simulink model "ALL_JP360_DBW_V6_5_1103"  (R2022a)
settings: Solver=FixedStepAuto  StartTime=0.0  StopTime=inf  FixedStep=0.01  RelTol=1e-3  EnableMultiTasking=on
model workspace (MAT data in the model file):
  g = 9.8
undefined symbols (not defined in the file or in its folder): canChannel, delta_v_p, IPM_Line_C0, IPM_Line_C1, IPM_Line_C2, IPM_Line_C3, M, M_p, MRR_ObjDistX, MRR_ObjDistY, MRR_ObjFusionCamID, MRR_ObjFusionSig, MRR_ObjID, MRR_ObjRelVelX, MRR_ObjRelVelY, MRR_ObjType, MRR_ObjUpdFlg, none, obj_vaild, untracktime, V, videoinput
libraries: canfdmsglib x230, canfdlib x76, slpidlib x24, simulink x18, dspstat3 x14, ctrlSharedLib x1, simulink_extras x1, imaqlib x1, realtime_pacer_lib x1, dspvision x1, visionsinks x1
(part 2 of 55)

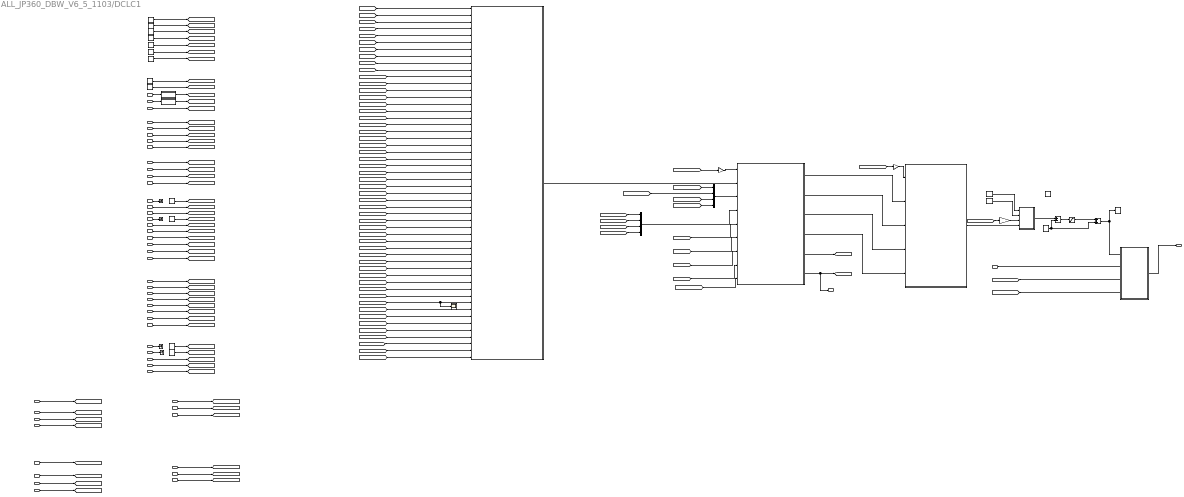
== system ALL_JP360_DBW_V6_5_1103/DCLC1 ==
  note: 0x0: Undecided 0x1: Solid实线 0x2: Road Edge道路边缘 0x3: Dashed虚线 0x4: Double 双线 0x5: Bott's Dots美国特有的凸点标线
  note: 0: OFF 1: PASSIVE/STANDBY 4: ACTIVE 5: ERROR
  note: 0: OFF 1: Passive 2: Stand-By 3: Active-Control 5: Override 6:Standstill 7:Failure
  note: 参数权重
  note: DCLC
      | 使能信号
  note: 刹车油门
      | 转向灯方向盘
  note: 自车速度、加速度
  note: 车道线
  note: 车道线系数
  note: 1V1R
  note: 左前
  note: 右前
  note: 左后
  note: 右后
  ACC_Enable : Inport
  LKA_Enable : Inport  Port=2
  DCLC_Enable : Inport  Port=3  OutDataTypeStr=boolean
  ESP_Algt : Inport  Port=4
  ESP_Alat : Inport  Port=5
  ABS_VehSpdLgt : Inport  Port=6  OutDataTypeStr=single
  ABS_VehSpdLat : Inport  Port=7
  Obj_Speed : Inport  Port=8  OutDataTypeStr=single
  FLR_ObjRelVel : Inport  Port=9
  FLR_OBJ1_Dx : Inport  Port=10
  FLR_OBJ1_Dy : Inport  Port=11
  FRR_ObjRelVel : Inport  Port=12
  FRR_SystemStatus : Inport  Port=13
  FRR_OBJ1_Dx : Inport  Port=14
  FRR_OBJ1_Dy : Inport  Port=15
  RRR_ObjRelVel : Inport  Port=16
  RRR_SystemStatus : Inport  Port=17
  RRR_OBJ1_Dx : Inport  Port=18
  RRR_OBJ1_Dy : Inport  Port=19
  RLR_ObjRelVel : Inport  Port=20
  RLR_OBJ1_Dx : Inport  Port=21
  RLR_OBJ1_Dy : Inport  Port=22
  EMS_BrkPedalStasus : Inport  Port=23
  EMS_AccRAWPedalRatio : Inport  Port=24
  BCM_TurnIndicatorSts : Inport  Port=25
  BCM_TurnIndicatorDig : Inport  Port=26
  EPS_TorsionBarTorque : Inport  Port=27  OutDataTypeStr=single
  IPM_SensorState : Inport  Port=28
  IPM_Line01_ColorClass : Inport  Port=29
  IPM_Line01_Type : Inport  Port=30
  IPM_Line01_C2 : Inport  Port=31  OutDataTypeStr=single
  IPM_Line02_ColorClass : Inport  Port=32
  IPM_Line02_Type : Inport  Port=33
  IPM_Line02_C2 : Inport  Port=34  OutDataTypeStr=single
  IPM_Line01_C0 : Inport  Port=35  OutDataTypeStr=single
  IPM_Line02_C0 : Inport  Port=36  OutDataTypeStr=single
  IPM_Line03_C0 : Inport  Port=37  OutDataTypeStr=single
  IPM_Line04_C0 : Inport  Port=38  OutDataTypeStr=single
  IPM_Line01_C1 : Inport  Port=39  OutDataTypeStr=single
  IPM_Line02_C1 : Inport  Port=40  OutDataTypeStr=single
  IPM_Line03_C1 : Inport  Port=41  OutDataTypeStr=single
  IPM_Line04_C1 : Inport  Port=42  OutDataTypeStr=single
  IPM_Line01_Existence_Probability : Inport  Port=43  OutDataTypeStr=single
  IPM_Line02_Existence_Probability : Inport  Port=44  OutDataTypeStr=single
  MRR_F_Object_dx : Inport  Port=45  OutDataTypeStr=single
  MRR_F_Object_dy : Inport  Port=46  OutDataTypeStr=single
  MRR_HWFail : Inport  Port=47
  IPM_Line03_Existence_Probability : Inport  Port=48  OutDataTypeStr=single
  IPM_Line04_Existence_Probability : Inport  Port=49  OutDataTypeStr=single
  SAS_SteerWheelAngle1 : Inport  Port=50
  Add : Sum  Inputs=+-
  Add1 : Sum
  AngleSaftyLimitedCal : MATLAB Function  TreatAsAtomicUnit=on
  Constant : Constant  Value=0.5  OutDataTypeStr=single
  Constant1 : Constant  Value=2.8  OutDataTypeStr=single
  Constant11 : Constant  Value=1.5  OutDataTypeStr=single
  Constant12 : Constant  Value=200  OutDataTypeStr=int32
  Constant13 : Constant  Value=100  OutDataTypeStr=single
  Constant2 : Constant
  Constant3 : Constant
  Constant{36..37,41,45} (4 alike) : Constant  OutDataTypeStr=single
  Constant4 : Constant  Value=100
  Constant48 : Constant  Value=130  OutDataTypeStr=single
  Constant49 : Constant  Value=20  OutDataTypeStr=single
  Constant5 : Constant  Value=150
  DCLC planner : Subsystem
  DCLC状态机 : Subsystem
  Data Store Memory : DataStoreMemory  DataStoreName=angle  ReadBeforeWriteMsg=warning  WriteAfterWriteMsg=warning  WriteAfterReadMsg=warning  ShowAdditionalParam=off  OutDataTypeStr=single
  Data Store Read : DataStoreRead  DataStoreName=angle  IndexOptions=Index vector (dialog)  Indices=1  OutputSizes=1
  Data Store Write : DataStoreWrite  DataStoreName=angle  IndexOptions=Index vector (dialog)  Indices=1  OutputSizes=1
  Gain1 : Gain  Gain=1/3.6
  Gain2 : Gain  Gain=1/3.6
  Gain3 : Gain  Gain=1/3.6
  LQR : Subsystem
  MATLAB Function : MATLAB Function  TreatAsAtomicUnit=on
  MATLAB Function1 : MATLAB Function  TreatAsAtomicUnit=on
  Mux : Mux
  Mux1 : Mux
  Saturation : Saturate  UpperLimit=0.1  LowerLimit=-0.1
  Scope : Scope
  Terminator{,1..3} (4 alike) : Terminator
  steering_angle_to_torque : Subsystem
  torque : Outport
  DCLC_status : Outport  Port=2
  wires:
  [ESP_Alat] -> DCLC状态机/10(ay)  "自车加速度 ay"
  FLR_OBJ1_Dy/1 -> [FLR_OBJ1_Dy]
  [FRR_ObjRelVel] -> DCLC状态机/6(右前车速度m/s)  "右前车速度m/s"
  [EPS_TorsionBarTorque] -> DCLC状态机/17(方向盘手力矩)  "方向盘手力矩"
  IPM_Line04_C1/1 -> [IPM_Line04_C1]
  Mux/1 -> DCLC planner/3(c0)  "c0"
  [FRR_OBJ1_Dy] -> DCLC状态机/42(与右前车的距离的y)  "与右前车的距离的y"
  [BCM_TurnIndicatorDig] -> DCLC状态机/16(转向灯故障)  "转向灯故障"
  [IPM_Line02_C2] -> DCLC状态机/49(右车道线曲率)  "左车道线的曲率"
  [ACC_Enable] -> DCLC状态机/45(ACC激活信号（暂定为1）)  "ACC激活信号（暂定为1）"
  [ABS_VehSpdLat] -> DCLC状态机/12(vy)  "自车速度 vy 暂定为0"
  [IPM_Line02_C0] -> DCLC状态机/24(后轴中心到右车道线的横向距离)  "后轴中心到右车道线的横向距离"
  DCLC planner/3(theta) -> LQR/4(thetar)  "theta"
  RRR_OBJ1_Dy/1 -> [RRR_OBJ1_Dy]
  EMS_AccRAWPedalRatio/1 -> [EMS_AccRAWPedalRatio]
  [t_lc] -> DCLC状态机/3(t_lc)  "t_lc"
  [IPM_Line04_C0] -> Mux/4
  [DCLC_Enable] -> DCLC状态机/43(DCLC开关)  "DCLC开关"
  RRR_ObjRelVel/1 -> [RRR_ObjRelVel]
  DCLC planner/5(reach_dest) -> [Reach_Destination]
  [DCLC_Speed_Upper] -> DCLC状态机/35(DCLC失效车速上限/km/h)  "DCLC失效车速上限/km/h"
  [ESP_Algt] -> DCLC状态机/9(ax)  "自车加速度 ax"
  [RLR_ObjRelVel] -> DCLC状态机/8(左后车速度m/s)  "左后车速度m/s"
  [IPM_Line03_C0] -> Mux/1
  [t_headway] -> DCLC状态机/1(t_headway)  "t_headway"
  [FRR_SystemStatus] -> DCLC状态机/19(右前雷达状态)  "右前雷达状态"
  IPM_Line02_Type/1 -> [IPM_Line02_Type]
  [IPM_Line01_Type] -> DCLC状态机/21(左车道线类型)  "左车道线类型"
  DCLC planner/2(yrr) -> LQR/3(yrr)  "yrr"
  RRR_SystemStatus/1 -> [RRR_SystemStatus]
  [IPM_Line01_Existence_Probability] -> DCLC状态机/37(左车道清晰状态（信号名暂不确定）)  "左车道清晰状态（信号名暂不确定）"
  [IPM_SensorState] -> DCLC状态机/25(摄像头状态)  "摄像头状态"
  LKA_Enable/1 -> MATLAB Function1/1(LKA_Enable)
  [ABS_VehSpdLgt] -> Gain2/1  "vx"
  [IPM_Line02_ColorClass] -> DCLC状态机/47(右车道线颜色)  "右车道线颜色"
  [Reach_Destination] -> Scope/1, DCLC状态机/44(换道结束标志（DCLC算法给出）)  "换道结束标志（DCLC算法给出）"
  [MRR_HWFail] -> DCLC状态机/28(1V1R雷达故障)  "1V1R雷达故障"
  [IPM_Line02_C1] -> Mux1/3
  DCLC planner/4(kr) -> LQR/5(kappar)  "kr"
  [FRR_OBJ1_Dx] -> DCLC状态机/41(与右前车的距离的x)  "与右前车的距离的x"
  DCLC状态机/1(dclc_sts) -> DCLC planner/2(dclc_sts)  "dclc_sts"
  [t_del] -> DCLC状态机/2(t_del)  "t_del"
  [BCM_TurnIndicatorSts] -> DCLC状态机/15(转向灯请求)  "转向灯请求"
  [lat_weight] -> DCLC planner/7(lat_weight)
  [IPM_Line01_ColorClass] -> DCLC状态机/20(左车道线颜色)  "左车道线颜色"
  [MRR_F_Object_dy] -> DCLC状态机/27(与前车的距离的y)  "与前车的距离的y"
  [EMS_AccRAWPedalRatio] -> DCLC状态机/14(油门信号有效性)  "油门信号有效性"
  [Obj_Speed] -> DCLC状态机/4(前车速度m/s)  "前车速度m/s"
  [IPM_Line01_C0] -> DCLC状态机/22(后轴中心到左车道线的横向距离)  "后轴中心到左车道线的横向距离"
  [RLR_OBJ1_Dx] -> DCLC状态机/29(与左后车的距离的x)  "与左后车的距离的x"
  [FLR_OBJ1_Dx] -> DCLC状态机/39(与左前车的距离的x)  "与左前车的距离的x"
  [RRR_OBJ1_Dx] -> DCLC状态机/32(与右后车的距离的x)  "与右后车的距离的x"
  BCM_TurnIndicatorSts/1 -> [BCM_TurnIndicatorSts]
  [ABS_VehSpdLgt] -> DCLC状态机/11(vx)  "自车速度 vx"
  [FRR_SystemStatus] -> DCLC状态机/18(左前雷达故障（用右前代替）)  "左前雷达故障（用右前代替）"
  [EMS_BrkPedalStasus] -> DCLC状态机/13(刹车信号有效性)  "刹车信号有效性"
  DCLC planner/1(xrr) -> LQR/2(xrr)  "xrr"
  [IPM_Line01_C0] -> Mux/2
  [MRR_F_Object_dx] -> DCLC状态机/26(与前车的距离的x)  "与前车的距离的x"
  [FLR_OBJ1_Dy] -> DCLC状态机/40(与左前车的距离的y)  "与左前车的距离的y"
  [pre_positio] -> DCLC planner/5(start_position)
  MRR_F_Object_dy/1 -> [MRR_F_Object_dy]
  [IPM_Line02_Existence_Probability] -> DCLC状态机/38(右车道清晰状态（信号名暂不确定）)  "右车道清晰状态（信号名暂不确定）"
  [LKA_Enable] -> DCLC状态机/46(LKA激活信号（暂定为1）)  "LKA激活信号（暂定为1）"
  [RLR_OBJ1_Dy] -> DCLC状态机/30(与左后车的距离的y)  "与左后车的距离的y"
  [DCLC_Speed_Lower] -> DCLC状态机/36(DCLC失效车速下限/km/h)  "DCLC失效车速下限/km/h"
  [RRR_SystemStatus] -> DCLC状态机/34(右后雷达状态)  "右后雷达状态"
  [RRR_ObjRelVel] -> DCLC状态机/7(右后车速度m/s)  "右后车速度m/s"
  [IPM_Line01_C2] -> DCLC状态机/23(左车道线的曲率)  "左车道线的曲率"
  [IPM_Line02_C0] -> Mux/3
  [RRR_SystemStatus] -> DCLC状态机/31(左后雷达失效（用右后雷达代替）)  "左后雷达失效（用右后雷达代替）"
  [IPM_Line03_C1] -> Mux1/1
  [IPM_Line01_C1] -> Mux1/2
  [IPM_Line04_C1] -> Mux1/4
  IPM_Line04_C0/1 -> [IPM_Line04_C0]
  [FLR_ObjRelVel] -> DCLC状态机/5(左前车速度m/s)  "左前车速度m/s"
  IPM_Line02_Existence_Probability/1 -> [IPM_Line02_Existence_Probability]
  Mux1/1 -> DCLC planner/4(C1)  "c1"
  [lon_weight] -> DCLC planner/6(lon_weight)
  [IPM_Line02_Type] -> DCLC状态机/48(右车道线类型)  "右车道线类型"
  [RRR_OBJ1_Dy] -> DCLC状态机/33(与右后车的距离的y)  "与右后车的距离的y"
  [change_time_weight] -> DCLC planner/8(change_time_weight)
  FRR_OBJ1_Dx/1 -> [FRR_OBJ1_Dx]
  FRR_ObjRelVel/1 -> [FRR_ObjRelVel]
  MRR_HWFail/1 -> [MRR_HWFail]
  FLR_ObjRelVel/1 -> [FLR_ObjRelVel]
  ABS_VehSpdLat/1 -> [ABS_VehSpdLat]
  IPM_Line01_C1/1 -> [IPM_Line01_C1]
  RLR_OBJ1_Dx/1 -> [RLR_OBJ1_Dx]
  FLR_OBJ1_Dx/1 -> [FLR_OBJ1_Dx]
  ACC_Enable/1 -> MATLAB Function/1(ACC_Enable)
  RLR_ObjRelVel/1 -> [RLR_ObjRelVel]
  FRR_OBJ1_Dy/1 -> [FRR_OBJ1_Dy]
  RRR_OBJ1_Dx/1 -> [RRR_OBJ1_Dx]
  RLR_OBJ1_Dy/1 -> [RLR_OBJ1_Dy]
  FRR_SystemStatus/1 -> [FRR_SystemStatus]
  IPM_Line01_Type/1 -> [IPM_Line01_Type]
  IPM_Line01_Existence_Probability/1 -> [IPM_Line01_Existence_Probability]
  IPM_Line01_C2/1 -> [IPM_Line01_C2]
  IPM_SensorState/1 -> [IPM_SensorState]
  ESP_Algt/1 -> [ESP_Algt]
  EPS_TorsionBarTorque/1 -> [EPS_TorsionBarTorque]
  IPM_Line02_C1/1 -> [IPM_Line02_C1]
  IPM_Line03_C1/1 -> [IPM_Line03_C1]
  ESP_Alat/1 -> [ESP_Alat]
  EMS_BrkPedalStasus/1 -> [EMS_BrkPedalStasus]
  IPM_Line02_C2/1 -> [IPM_Line02_C2]
  IPM_Line03_C0/1 -> [IPM_Line03_C0]
  IPM_Line01_C0/1 -> [IPM_Line01_C0]
  DCLC_Enable/1 -> [DCLC_Enable]
  IPM_Line02_C0/1 -> [IPM_Line02_C0]
  BCM_TurnIndicatorDig/1 -> [BCM_TurnIndicatorDig]
  LQR/1(steering_angle) -> AngleSaftyLimitedCal/4(angle)  "steering_angle"
  Constant/1 -> AngleSaftyLimitedCal/1(a)
  Constant1/1 -> AngleSaftyLimitedCal/2(L)
  [ABS_VehSpdLgt] -> Gain3/1  "vx"
  [ABS_VehSpdLgt] -> Gain1/1
  Gain3/1 -> AngleSaftyLimitedCal/3(V)
  Data Store Read/1 -> Add/2, Add1/2
  Add/1 -> Saturation/1
  Add1/1 -> Data Store Write/1, steering_angle_to_torque/1(desire_steering_angle)
  DCLC planner/6(status) -> DCLC_status/1, [Pass_Midline]
  [Pass_Midline] -> DCLC状态机/50(变道越过车道线标志)  "变道越过车道线标志（1表示未越过车道线，2表示越过车道线）"
  ABS_VehSpdLgt/1 -> [ABS_VehSpdLgt]
  Gain2/1 -> DCLC planner/1(vx)
  Gain1/1 -> LQR/1(vx)
  Constant41/1 -> [t_del]
  Constant12/1 -> [pre_positio]
  Constant36/1 -> [lon_weight]
  Constant13/1 -> [lat_weight]
  Constant37/1 -> [change_time_weight]
  Constant45/1 -> [t_lc]
  Constant11/1 -> [t_headway]
  Constant49/1 -> [DCLC_Speed_Lower]
  Constant48/1 -> [DCLC_Speed_Upper]
  IPM_Line01_ColorClass/1 -> Terminator/1
  Constant2/1 -> [IPM_Line01_ColorClass]
  IPM_Line02_ColorClass/1 -> Terminator1/1
  Constant3/1 -> [IPM_Line02_ColorClass]
  Obj_Speed/1 -> Terminator2/1
  Constant4/1 -> [Obj_Speed]
  MATLAB Function/1(u) -> [ACC_Enable]
  MATLAB Function1/1(u) -> [LKA_Enable]
  IPM_Line03_Existence_Probability/1 -> [IPM_Line03_Existence_Probability]
  IPM_Line04_Existence_Probability/1 -> [IPM_Line04_Existence_Probability]
  [IPM_Line03_Existence_Probability] -> DCLC状态机/51(leftleft_line_pro)  "左左车道线清晰状态"
  [IPM_Line04_Existence_Probability] -> DCLC状态机/52(rightright_line_pro)  "右右车道线清晰状态"
  MRR_F_Object_dx/1 -> Terminator3/1
  Constant5/1 -> [MRR_F_Object_dx]
  AngleSaftyLimitedCal/1(angle_limited) -> Add/1
  Saturation/1 -> Add1/1
  [ABS_VehSpdLgt] -> steering_angle_to_torque/3(vx km/h)
  SAS_SteerWheelAngle1/1 -> steering_angle_to_torque/2(acture_steering_angle)
  [ABS_VehSpdLat] -> steering_angle_to_torque/4(vy km/h)
  steering_angle_to_torque/1(torque) -> torque/1
  [BCM_TurnIndicatorSts] -> DCLC planner/9(turn_request)  "转向灯请求"

== system ALL_JP360_DBW_V6_5_1103/Error ==

== system ALL_JP360_DBW_V6_5_1103/LKA_Control ==
  note: 0: OFF
      | 1: Passive
      | 2: Stand-By
      | 3: Active-Control
      | 5: Override
      | 6: Standstill
      | 7: Failure
  note: Lane_status:
      | 0：无车道线
      | 1：单车道线
      | 2：双车道线
      | 3：骑线
  SWM : Inport
  SWM_TurnIndicatorAct : Inport  Port=2
  ESP_YawRateStatus : Inport  Port=3
  ABS_VehSpdLgtStatus : Inport  Port=4
  ESP_Master_Cylinder_Pressure : Inport  Port=5
  SRS_SBR_Driver : Inport  Port=6
  MRR_HWFail : Inport  Port=7
  IPM_SensorState : Inport  Port=8
  TCU_GearSelectorReq : Inport  Port=9
  SAS_SteerWheelRotSpd : Inport  Port=10
  EPS_TorsionBarTorque : Inport  Port=11
  ESP_EspCtrlActv : Inport  Port=12
  EMS_IndicatedEngError : Inport  Port=13
  BCM_DoorStsFrntLe : Inport  Port=14
  BCM_DoorStsRearRi : Inport  Port=15
  BCM_DoorStsFrntRi : Inport  Port=16
  BCM_DoorStsRearLe : Inport  Port=17
  BCM_EnginehoodSts : Inport  Port=18
  ESP_YawRate : Inport  Port=19
  ABS_VehSpdLgt : Inport  Port=20
  ABS_AbsCtrlActv : Inport  Port=21
  SAS_SteerWheelAngle : Inport  Port=22
  SAS_SteerWheelRotSpdStatus : Inport  Port=23
  EPS_LKAControlStatus : Inport  Port=24
  EPS_LKAResponseTorque : Inport  Port=25
  EPS_EPSPAMSts : Inport  Port=26
  ESP_EspEnableSts : Inport  Port=27
  ESP_Master_Cylinder_Pressure_Status : Inport  Port=28
  IPM_Line01_C0 : Inport  Port=29
  IPM_Line01_C1 : Inport  Port=30
  IPM_Line01_C2 : Inport  Port=31
  IPM_Line01_C3 : Inport  Port=32
  IPM_Line02_C0 : Inport  Port=33
  IPM_Line02_C1 : Inport  Port=34
  IPM_Line02_C2 : Inport  Port=35
  IPM_Line02_C3 : Inport  Port=36
  IPM_Line01_Existence_Probability : Inport  Port=37
  IPM_Line02_Existence_Probability : Inport  Port=38
  acc_sta : Inport  Port=39
  DCLC_Status : Inport  Port=40
  Chart : Stateflow chart  TreatAsAtomicUnit=on
  Constant : Constant  Value=0  OutDataTypeStr=int8
  Constant1 : Constant  Value=3  OutDataTypeStr=single
  Constant3 : Constant  Value=0  OutDataTypeStr=int8
  Constant5 : Constant  OutDataTypeStr=int8
  Data Type Conversion : DataTypeConversion  OutDataTypeStr=single  SaturateOnIntegerOverflow=off  RndMeth=Floor
  Data Type Conversion3 : DataTypeConversion  OutDataTypeStr=int8  SaturateOnIntegerOverflow=off  RndMeth=Floor
  Display{,1..4} (5 alike) : Display
  LKA_Cal : Subsystem
  Lane_Status : Subsystem
  Mux1 : Mux  Inputs=8
  Scope : Scope  NumInputPorts=2
  To Workspace : ToWorkspace  VariableName=L_status  SaveFormat=Timeseries  SampleTime=-1
  To Workspace1 : ToWorkspace  VariableName=LKA_status  SaveFormat=Structure With Time  SampleTime=-1
  To Workspace2 : ToWorkspace  VariableName=TorsionBar_tor  SaveFormat=Structure With Time  SampleTime=-1
  To Workspace3 : ToWorkspace  VariableName=C  SaveFormat=Structure With Time  SampleTime=-1
  To Workspace4 : ToWorkspace  VariableName=L1_pro  SaveFormat=Structure With Time  SampleTime=-1
  To Workspace5 : ToWorkspace  VariableName=L2_pro  SaveFormat=Structure With Time  SampleTime=-1
  LKAReq_angle : Outport
  IPM_LineAssit_Status : Outport  Port=2
  err_now : Outport  Port=3
  wires:
  ESP_Master_Cylinder_Pressure_Status/1 -> Chart/33(ESP_Master_Cylinder_Pressure_Status)
  BCM_DoorStsRearLe/1 -> Chart/20(BCM_DoorStsRearLe)
  ESP_EspCtrlActv/1 -> Chart/26(ESP_EspCtrlActv)
  EPS_EPSPAMSts/1 -> Chart/29(EPS_EPSPAMSts)
  [ABS_VehSpdLgt] -> LKA_Cal/4(ABS_Vhlspd)
  SRS_SBR_Driver/1 -> Chart/21(SRS_SBR_Driver)
  BCM_DoorStsFrntRi/1 -> Chart/19(BCM_DoorStsFrntRi)
  [C2] -> Chart/9(LaneCurvature)
  BCM_DoorStsFrntLe/1 -> Chart/17(BCM_DoorStsFrntLe)
  EPS_TorsionBarTorque/1 -> To Workspace2/1, Chart/24(EPS_TorsionBarTorque), Display/1
  EPS_LKAResponseTorque/1 -> Chart/28(EPS_LKAResponseTorque)
  EPS_LKAControlStatus/1 -> Chart/25(EPS_LKAControlStatus)
  EMS_IndicatedEngError/1 -> Chart/30(EMS_IndicatedEngError)
  Data Type Conversion3/1 -> Chart/5(ESP_YawRateStatus)
  Constant5/1 -> Chart/2(IPM_LineAssit_LeftVisualization), Chart/3(IPM_LineAssit_RightVisualization)
  TCU_GearSelectorReq/1 -> Chart/23(TCU_GearSelectorReq)
  SAS_SteerWheelRotSpd/1 -> Chart/27(SAS_SteerWheelRotSpd)
  ESP_YawRateStatus/1 -> Data Type Conversion3/1
  ESP_YawRate/1 -> Chart/6(ESP_YawRate)
  BCM_DoorStsRearRi/1 -> Chart/18(BCM_DoorStsRearRi)
  BCM_EnginehoodSts/1 -> Chart/22(BCM_EnginehoodSts)
  SAS_SteerWheelRotSpdStatus/1 -> Chart/32(SAS_SteerWheelRotSpdStatus)
  Constant3/1 -> Chart/11(LaneChange)
  IPM_SensorState/1 -> Chart/14(IPM_SensorState)
  Chart/1(IPM_LineAssit_Status) -> Display3/1, To Workspace1/1, Scope/2, [LKA_status], IPM_LineAssit_Status/1  "LKA"
  ABS_AbsCtrlActv/1 -> Chart/12(ABS_AbsCtrlActv)
  SAS_SteerWheelAngle/1 -> LKA_Cal/3(SAS_SteerWheelAngle), Display2/1
  ESP_EspEnableSts/1 -> Chart/31(ESP_EspEnableSts)
  MRR_HWFail/1 -> Chart/13(MRR_HWFail)
  ABS_VehSpdLgt/1 -> Data Type Conversion/1, [ABS_VehSpdLgt]
  ABS_VehSpdLgtStatus/1 -> Chart/7(ABS_VehSpdLgtStatus)
  Constant/1 -> Chart/15(lka_state_sw)
  Data Type Conversion/1 -> Chart/8(ABS_VehSpdLgt)
  [Ct] -> LKA_Cal/1(Ct)
  Constant1/1 -> Chart/10(LaneWidth)
  ESP_Master_Cylinder_Pressure/1 -> Chart/16(ESP_Master_Cylinder_Pressure)
  SWM/1 -> Chart/1(LKASwitch)
  IPM_Line01_Existence_Probability/1 -> Lane_Status/2(IPM_Line01_Existence_Probability), To Workspace4/1
  IPM_Line02_Existence_Probability/1 -> Lane_Status/3(IPM_Line02_Existence_Probability), To Workspace5/1
  Lane_Status/1(Ct) -> [Ct]
  Lane_Status/2(lane_status) -> Scope/1, [Lane_status], Display1/1, To Workspace/1  "lane"
  [Lane_status] -> Chart/34(Lane_status)
  SWM_TurnIndicatorAct/1 -> Chart/4(SWM_TurnIndicationAct)
  LKA_Cal/1(LKAReq_angle) -> LKAReq_angle/1, Display4/1
  DCLC_Status/1 -> Chart/35(DCLC_Status)
  acc_sta/1 -> Chart/36(acc_sta)
  Lane_Status/3(ang) -> [ang]
  [ang] -> Chart/37(degre)
  LKA_Cal/2(err_now) -> err_now/1
  [LKA_status] -> LKA_Cal/2(LKA_status)
  Lane_Status/4(C2) -> [C2]
  Mux1/1 -> Lane_Status/1(LRC), To Workspace3/1
  IPM_Line01_C0/1 -> Mux1/1
  IPM_Line01_C1/1 -> Mux1/2
  IPM_Line01_C2/1 -> Mux1/3
  IPM_Line02_C0/1 -> Mux1/5
  IPM_Line02_C1/1 -> Mux1/6
  IPM_Line01_C3/1 -> Mux1/4
  IPM_Line02_C2/1 -> Mux1/7
  IPM_Line02_C3/1 -> Mux1/8

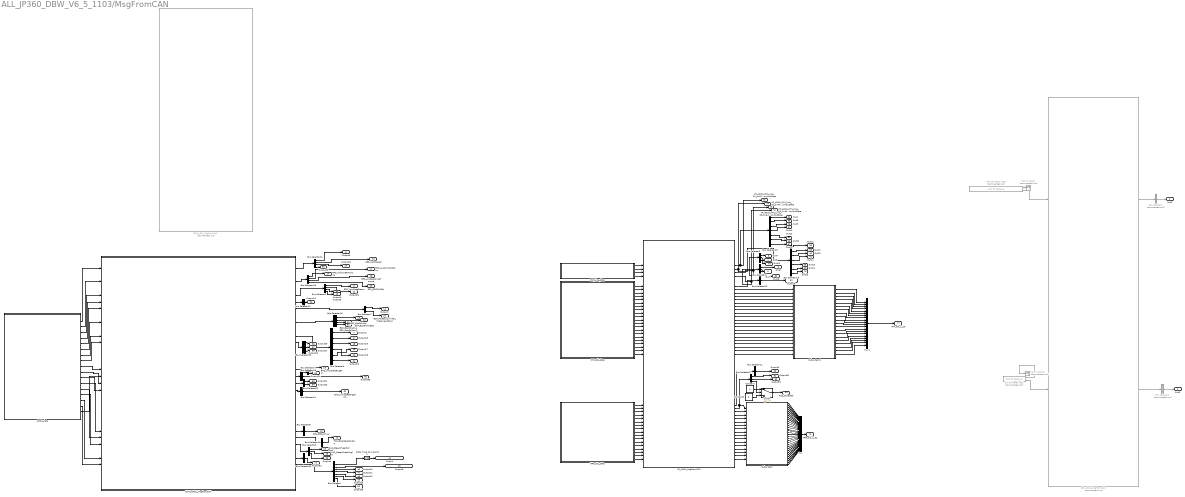
== system ALL_JP360_DBW_V6_5_1103/MsgFromCAN ==
  ADCU_data : Subsystem
  Bus Selector : BusSelector  OutputSignals=SWM_LaneAssistSwitch,SWM_ACCResume,SWM_ACCSet,SWM_ACCSwitch,SWM_ACCvSetPlus,SWM_ACCvSetMinus,SWM_ACCtauGapSetMinus
  Bus Selector1 : BusSelector  Commented=on  OutputSignals=FRR_SystemStatus
  Bus Selector10 : BusSelector  OutputSignals=IPM_SensorState
  Bus Selector11 : BusSelector  OutputSignals=MRR_HWFail
  Bus Selector12 : BusSelector  OutputSignals=ABS_VehSpdLgtStatus,ABS_VehSpdLgt,ABS_AbsCtrlActv,ABS_VehSpdDirection
  Bus Selector13 : BusSelector  OutputSignals=IPM_Line01_C0,IPM_Line01_C1,IPM_Line01_C2,IPM_Line01_C3,IPM_Line01_Type,IPM_Line01_ColorClass,IPM_Line01_Existence_Probability
  Bus Selector14 : BusSelector  OutputSignals=TCU_GearSelectorReq
  Bus Selector15 : BusSelector  OutputSignals=EPS_TorsionBarTorque,EPS_LKAControlStatus,EPS_LKAResponseTorque,EPS_EPSPAMSts
  Bus Selector16 : BusSelector  OutputSignals=ESP_EspCtrlActv,ESP_EspEnableSts,ESP_EPBStatus,ESP_AvhActive
  Bus Selector17 : BusSelector  OutputSignals=EMS_IndicatedEngError,EMS_IndicatedDriverOverride
  Bus Selector18 : BusSelector  OutputSignals=IPM_Line02_C0,IPM_Line02_C1,IPM_Line02_C2,IPM_Line02_C3,IPM_Line02_Type,IPM_Line02_ColorClass,IPM_Line02_Existence_Probability
  Bus Selector19 : BusSelector  OutputSignals=EMS_IndicatedRealEngTorq
  Bus Selector2 : BusSelector  Commented=on  OutputSignals=RRR_SystemStatus
  Bus Selector21 : BusSelector  OutputSignals=ESP_VehicleStandstill
  Bus Selector22 : BusSelector  OutputSignals=EMS_AccRAWPedalRatio,EMS_BrkPedalStasus
  Bus Selector23 : BusSelector  OutputSignals=BCM_PowerModeInvalid,BCM_PowerMode,BCM_Mechanical_Hand_Brake
  Bus Selector24 : BusSelector  OutputSignals=IC_VehSpd_HMI
  Bus Selector27 : BusSelector  OutputSignals=MRR_ObjDistX_01,MRR_ObjRelVelX_01,MRR_ObjType_01
  Bus Selector28 : BusSelector  OutputSignals=SWM_TurnIndicationAct
  Bus Selector3 : BusSelector  OutputSignals=IPM_Line03_C0,IPM_Line03_C1,IPM_Line03_Existence_Probability
  Bus Selector4 : BusSelector  OutputSignals=IPM_Line04_C0,IPM_Line04_C1,IPM_Line04_Existence_Probability
  Bus Selector5 : BusSelector  OutputSignals=ESP_YawRateStatus,ESP_YawRate,ESP_Alat,ESP_Algt
  Bus Selector6 : BusSelector  OutputSignals=BCM_TurnIndicatorSts,BCM_DoorStsFrntLe,BCM_DoorStsRearRi,BCM_DoorStsRearLe,BCM_DoorStsFrntRi,BCM_EnginehoodSts
  Bus Selector7 : BusSelector  OutputSignals=ESP_Master_Cylinder_Pressure,ESP_Master_Cylinder_Pressure_Status
  Bus Selector8 : BusSelector  OutputSignals=SRS_SBR_Driver
  Bus Selector9 : BusSelector  OutputSignals=SAS_SteerWheelRotSpd,SAS_SteerWheelAngle,SAS_SteerWheelRotSpdStatus
  CAN FD Receive50 : canfdlib/CAN FD Receive  Commented=on  BlockHandle=78400.0006  Device=MathWorks Virtual 1 (Channel 1)  ObjConstructor=canChannel('MathWorks', 'Virtual 1', 1, 'ProtocolMode', 'CAN FD')  EnableStandardIDsFilter=off  StdIDsCombo=Allow only  StandardIDs=114  EnableExtendedIDsFilter=off  ExtIDsCombo=Allow all  ExtendedIDs=0  SampleTime=0.01  MsgsPerTimestep=all  InternalFilterUpdateStatus=on  BusOutput=on
      settings: SourceProductBaseCode=VN
  CAN FD Receive51 : canfdlib/CAN FD Receive  Commented=on  BlockHandle=78403.0004  Device=MathWorks Virtual 1 (Channel 1)  ObjConstructor=canChannel('MathWorks', 'Virtual 1', 1, 'ProtocolMode', 'CAN FD')  EnableStandardIDsFilter=off  StdIDsCombo=Allow only  StandardIDs=115  EnableExtendedIDsFilter=off  ExtIDsCombo=Allow all  ExtendedIDs=0  SampleTime=0.01  MsgsPerTimestep=all  InternalFilterUpdateStatus=on  BusOutput=on
      settings: SourceProductBaseCode=VN
  CCAN_ADCU_MsgFromCAN : Subsystem
  CCAN_GW_MsgFromCAN : Subsystem  Commented=on
  Constant : Constant  OutDataTypeStr=boolean
  Constant1 : Constant  Value=0  OutDataTypeStr=boolean
  Data Type Conversion1 : DataTypeConversion  OutDataTypeStr=int8  SaturateOnIntegerOverflow=off  RndMeth=Floor
  IPM_Line_data : Subsystem
  IPM_Obj_data : Subsystem
  MRR_Obj_data : Subsystem
  Mux : Mux  Inputs=32
  Mux1 : Mux  Inputs=20
  SRR_ADCU_MsgFromCAN : Subsystem  Commented=on
  Subsystem : Subsystem
  Subsystem1 : Subsystem
  Switch : Switch  Criteria=u2 > Threshold  SaturateOnIntegerOverflow=off  InputSameDT=off
  Terminator22 : Terminator  Commented=on
  Terminator23 : Terminator  Commented=on
  VR_ADCU_MsgFromCAN : Subsystem
  Out2 : Outport
  Out3 : Outport  Port=2
  Out4 : Outport  Port=3
  Out5 : Outport  Port=4
  Out6 : Outport  Port=5
  Out7 : Outport  Port=6
  Output1 : Outport  Port=7
  ESP_YawRateStatus : Outport  Port=8
  Output3 : Outport  Port=9
  SRS_SBR_Driver : Outport  Port=10
  Output7 : Outport  Port=11
  TCU_GearSelectorReq : Outport  Port=12
  SAS_SteerWheelRotSpd : Outport  Port=13
  EPS_TorsionBarTorque : Outport  Port=14
  ESP_EspCtrlActv : Outport  Port=15
  EMS_IndicatedEngError : Outport  Port=16
  Output15 : Outport  Port=17
  Output16 : Outport  Port=18
  Output17 : Outport  Port=19
  Output18 : Outport  Port=20
  Output19 : Outport  Port=21
  Output20 : Outport  Port=22
  ABS_VehSpdLgt : Outport  Port=23
  Output22 : Outport  Port=24
  SAS_SteerWheelAngle : Outport  Port=25
  Output4 : Outport  Port=26
  EPS_LKAControlStatus : Outport  Port=27
  EPS_LKAResponseTorque : Outport  Port=28
  EPS_EPSPAMSts : Outport  Port=29
  ESP_EspEnableSts : Outport  Port=30
  ESP_Master_Cylinder_Pressure_Status : Outport  Port=31
  Output6 : Outport  Port=32
  Output5 : Outport  Port=33
  Out1 : Outport  Port=34
  Out8 : Outport  Port=35
  Out9 : Outport  Port=36
  Out10 : Outport  Port=37
  Out11 : Outport  Port=38
  Out12 : Outport  Port=39
  Out13 : Outport  Port=40
  Out14 : Outport  Port=41
  Output2 : Outport  Port=42
  Output8 : Outport  Port=43
  Output : Outport  Port=44
  Output9 : Outport  Port=45
  Output10 : Outport  Port=46
  Output11 : Outport  Port=47
  Output12 : Outport  Port=48
  Output13 : Outport  Port=49
  Output14 : Outport  Port=50
  ESP_EspCtrlActv1 : Outport  Port=51
  ESP_EspCtrlActv2 : Outport  Port=52
  Output21 : Outport  Port=53
  Output23 : Outport  Port=54
  Output24 : Outport  Port=55
  Output25 : Outport  Port=56
  Output26 : Outport  Port=57
  Output27 : Outport  Port=58
  Output28 : Outport  Port=59
  Output29 : Outport  Port=60
  EMS_IndicatedEngError1 : Outport  Port=61
  Output30 : Outport  Port=62
  Output31 : Outport  Port=63
  ACC_Objected : Outport  Port=64
  Out20 : Outport  Port=65
  Out21 : Outport  Port=66
  Out22 : Outport  Port=67
  Out23 : Outport  Port=68
  Out24 : Outport  Port=69
  Out25 : Outport  Port=70
  Output32 : Outport  Port=71
  MRR_obj_1_32 : Outport  Port=72
  VR_ADCU_IPM_Line_01_0x640FromOutData : Outport  Port=73
  VR_ADCU_IPM_Line_02_0x641FromOutData : Outport  Port=74
  VR_ADCU_IPM_Line_03_0x642FromOutData : Outport  Port=75
  VR_ADCU_IPM_Line_04_0x643FromOutData : Outport  Port=76
  IPM_obj_1_20 : Outport  Port=77
  Output33 : Outport  Port=78
  Out15 : Outport  Port=79
  Out16 : Outport  Port=80
  wires:
  SRR_ADCU_MsgFromCAN/22(SRR_ADCU_FRR_AssistSysSt_0x72FromOutData) -> Bus Selector1/1  "SRR_ADCU_FRR_AssistSysSt_0x72FromOutData"
  Bus Selector1/1 -> Out2/1  "<FRR_SystemStatus>"
  Bus Selector2/1 -> Out3/1  "<RRR_SystemStatus>"
  SRR_ADCU_MsgFromCAN/64(SRR_ADCU_RRR_AssistSysSt_0x73FromOutData) -> Bus Selector2/1  "SRR_ADCU_FRR_AssistSysSt_0x72FromOutData"
  VR_ADCU_MsgFromCAN/8(VR_ADCU_IPM_Line_03_0x642FromOutData) -> VR_ADCU_IPM_Line_03_0x642FromOutData/1, Bus Selector3/1  "VR_ADCU_IPM_Line_03_0x642FromOutData"
  VR_ADCU_MsgFromCAN/9(VR_ADCU_IPM_Line_04_0x643FromOutData) -> Bus Selector4/1, VR_ADCU_IPM_Line_04_0x643FromOutData/1  "VR_ADCU_IPM_Line_04_0x643FromOutData"
  Bus Selector4/1 -> Out6/1  "<IPM_Line04_C0>"
  Bus Selector4/2 -> Out7/1  "<IPM_Line04_C1>"
  Bus Selector3/1 -> Out4/1  "<IPM_Line03_C0>"
  Bus Selector3/2 -> Out5/1  "<IPM_Line03_C1>"
  Bus Selector7/1 -> Output7/1  "<ESP_Master_Cylinder_Pressure>"
  Bus Selector5/2 -> Output20/1  "<ESP_YawRate>"
  Bus Selector7/2 -> ESP_Master_Cylinder_Pressure_Status/1  "<ESP_Master_Cylinder_Pressure_Status>"
  Bus Selector17/1 -> EMS_IndicatedEngError/1  "<EMS_IndicatedEngError>"
  Bus Selector16/2 -> ESP_EspEnableSts/1  "<ESP_EspEnableSts>"
  Bus Selector8/1 -> SRS_SBR_Driver/1  "<SRS_SBR_Driver>"
  Bus Selector12/1 -> Output3/1  "<ABS_VehSpdLgtStatus>"
  Bus Selector15/4 -> EPS_EPSPAMSts/1  "<EPS_EPSPAMSts>"
  CCAN_ADCU_MsgFromCAN/1(CCAN_ADCU_ABS_Sts_0x221FromOutData) -> Bus Selector12/1  "CCAN_ADCU_ABS_Sts_0x221FromOutData"
  Bus Selector9/2 -> SAS_SteerWheelAngle/1  "<SAS_SteerWheelAngle>"
  Bus Selector12/3 -> Output22/1  "<ABS_AbsCtrlActv>"
  CCAN_ADCU_MsgFromCAN/9(CCAN_ADCU_ESP_Status_0x243FromOutData) -> Bus Selector16/1  "CCAN_ADCU_ESP_Status_0x243FromOutData"
  CCAN_ADCU_MsgFromCAN/27(CCAN_ADCU_SAS_Sensor_0x175FromOutData) -> Bus Selector9/1  "CCAN_ADCU_SAS_Sensor_0x175FromOutData"
  Bus Selector6/4 -> Output18/1  "<BCM_DoorStsRearLe>"
  CCAN_ADCU_MsgFromCAN/7(CCAN_ADCU_ESP_Pressure_0x241FromOutData) -> Bus Selector7/1  "CCAN_ADCU_ESP_Pressure_0x241FromOutData"
  CCAN_ADCU_MsgFromCAN/25(CCAN_ADCU_GW_SRS_0x350FromOutData) -> Bus Selector8/1  "CCAN_ADCU_GW_SRS_0x350FromOutData"
  Bus Selector15/3 -> EPS_LKAResponseTorque/1  "<EPS_LKAResponseTorque>"
  Bus Selector6/2 -> Output15/1  "<BCM_DoorStsFrntLe>"
  Bus Selector6/1 -> Output1/1  "<BCM_TurnIndicatorSts>"
  Bus Selector6/6 -> Output19/1  "<BCM_EnginehoodSts>"
  Bus Selector/1 -> Data Type Conversion1/1  "<SWM_LaneAssistSwitch>"
  CCAN_ADCU_MsgFromCAN/26(CCAN_ADCU_GW_TCU_GearInfo_0x123FromOutData) -> Bus Selector14/1  "CCAN_ADCU_GW_TCU_GearInfo_0x123FromOutData"
  CCAN_ADCU_MsgFromCAN/30(CCAN_ADCU_SWM_MRR_0x31BFromOutData) -> Bus Selector/1  "CCAN_ADCU_SWM_MRR_0x31BFromOutData"
  CCAN_ADCU_MsgFromCAN/16(CCAN_ADCU_GW_EMS_TqWhl_0x111FromOutData) -> Bus Selector17/1  "CCAN_ADCU_GW_EMS_TqWhl_0x111FromOutData"
  Bus Selector15/1 -> EPS_TorsionBarTorque/1  "<EPS_TorsionBarTorque>"
  Bus Selector15/2 -> EPS_LKAControlStatus/1  "<EPS_LKAControlStatus>"
  Bus Selector5/1 -> ESP_YawRateStatus/1  "<ESP_YawRateStatus>"
  Bus Selector9/1 -> SAS_SteerWheelRotSpd/1  "<SAS_SteerWheelRotSpd>"
  CCAN_ADCU_MsgFromCAN/5(CCAN_ADCU_ESP_AxAy_0x242FromOutData) -> Bus Selector5/1  "CCAN_ADCU_ESP_AxAy_0x242FromOutData"
  CCAN_ADCU_MsgFromCAN/11(CCAN_ADCU_GW_BCM_Door_0x310FromOutData) -> Bus Selector6/1  "CCAN_ADCU_GW_BCM_Door_0x310FromOutData"
  Bus Selector6/5 -> Output17/1  "<BCM_DoorStsFrntRi>"
  Bus Selector12/2 -> ABS_VehSpdLgt/1  "<ABS_VehSpdLgt>"
  Bus Selector14/1 -> TCU_GearSelectorReq/1  "<TCU_GearSelectorReq>"
  Bus Selector6/3 -> Output16/1  "<BCM_DoorStsRearRi>"
  Bus Selector16/1 -> ESP_EspCtrlActv/1  "<ESP_EspCtrlActv>"
  CCAN_ADCU_MsgFromCAN/3(CCAN_ADCU_EPS_Advanced_0x176FromOutData) -> Bus Selector15/1  "CCAN_ADCU_EPS_Advanced_0x176FromOutData"
  Bus Selector10/1 -> Output6/1  "<IPM_SensorState>"
  VR_ADCU_MsgFromCAN/12(VR_ADCU_IPM_ObjHeader_0x630FromOutData) -> Bus Selector10/1  "VR_ADCU_IPM_ObjHeader_0x630FromOutData"
  Bus Selector11/1 -> Output5/1  "<MRR_HWFail>"
  VR_ADCU_MsgFromCAN/47(VR_ADCU_MRR_ObjHeader_0x680FromOutData) -> Bus Selector11/1  "VR_ADCU_MRR_ObjHeader_0x680FromOutData"
  VR_ADCU_MsgFromCAN/6(VR_ADCU_IPM_Line_01_0x640FromOutData) -> VR_ADCU_IPM_Line_01_0x640FromOutData/1, Bus Selector13/1  "VR_ADCU_IPM_Line_01_0x640FromOutData"
  VR_ADCU_MsgFromCAN/7(VR_ADCU_IPM_Line_02_0x641FromOutData) -> VR_ADCU_IPM_Line_02_0x641FromOutData/1, Bus Selector18/1  "VR_ADCU_IPM_Line_02_0x641FromOutData"
  Bus Selector13/1 -> Out1/1  "<IPM_Line01_C0>"
  Bus Selector13/2 -> Out8/1  "<IPM_Line01_C1>"
  Bus Selector13/3 -> Out9/1  "<IPM_Line01_C2>"
  Bus Selector13/4 -> Out10/1  "<IPM_Line01_C3>"
  Bus Selector18/1 -> Out11/1  "<IPM_Line02_C0>"
  Bus Selector18/2 -> Out12/1  "<IPM_Line02_C1>"
  Bus Selector18/3 -> Out13/1  "<IPM_Line02_C2>"
  Bus Selector18/4 -> Out14/1  "<IPM_Line02_C3>"
  Bus Selector9/3 -> Output4/1  "<SAS_SteerWheelRotSpdStatus>"
  Bus Selector5/3 -> Output2/1  "<ESP_Alat>"
  Bus Selector5/4 -> Output8/1  "<ESP_Algt>"
  Bus Selector/2 -> Output9/1  "<SWM_ACCResume>"
  Bus Selector/3 -> Output10/1  "<SWM_ACCSet>"
  Bus Selector/4 -> Output11/1  "<SWM_ACCSwitch>"
  Bus Selector/5 -> Output12/1  "<SWM_ACCvSetPlus>"
  Bus Selector/6 -> Output13/1  "<SWM_ACCvSetMinus>"
  CCAN_ADCU_MsgFromCAN/6(CCAN_ADCU_ESP_Direction_0x235FromOutData) -> Bus Selector21/1  "CCAN_ADCU_ESP_Direction_0x235FromOutData"
  Bus Selector21/1 -> Output14/1  "<ESP_VehicleStandstill>"
  Bus Selector16/4 -> ESP_EspCtrlActv2/1  "<ESP_AvhActive>"
  Bus Selector16/3 -> ESP_EspCtrlActv1/1  "<ESP_EPBStatus>"
  CCAN_ADCU_MsgFromCAN/18(CCAN_ADCU_GW_EMS_WhlTq_0x107FromOutData) -> Bus Selector22/1  "CCAN_ADCU_GW_EMS_WhlTq_0x107FromOutData"
  Bus Selector22/1 -> Output21/1  "<EMS_AccRAWPedalRatio>"
  Bus Selector22/2 -> Output23/1  "<EMS_BrkPedalStasus>"
  Bus Selector17/2 -> Output24/1  "<EMS_IndicatedDriverOverride>"
  CCAN_ADCU_MsgFromCAN/12(CCAN_ADCU_GW_Body_0x321FromOutData) -> Bus Selector23/1  "CCAN_ADCU_GW_Body_0x321FromOutData"
  Bus Selector23/1 -> Output25/1  "<BCM_PowerModeInvalid>"
  Bus Selector23/2 -> Output26/1  "<BCM_PowerMode>"
  Bus Selector23/3 -> Output27/1  "<BCM_Mechanical_Hand_Brake>"
  Bus Selector12/4 -> Output28/1  "<ABS_VehSpdDirection>"
  Bus Selector/7 -> Output29/1  "<SWM_ACCtauGapSetMinus>"
  CAN FD Receive50/1 -> Terminator22/1
  CAN FD Receive50/2 -> SRR_ADCU_MsgFromCAN/22(SRR_ADCU_FRR_AssistSysSt_0x72FromInData)
  CAN FD Receive51/2 -> SRR_ADCU_MsgFromCAN/64(SRR_ADCU_RRR_AssistSysSt_0x73FromInData)
  CAN FD Receive51/1 -> Terminator23/1
  CCAN_ADCU_MsgFromCAN/19(CCAN_ADCU_GW_IC_0x510FromOutData) -> Bus Selector24/1  "CCAN_ADCU_GW_IC_0x510FromOutData"
  Bus Selector24/1 -> EMS_IndicatedEngError1/1  "<IC_VehSpd_HMI>"
  VR_ADCU_MsgFromCAN/48(VR_ADCU_MRR_Obj_01_02_0x690FromOutData) -> Subsystem/1(VR_ADCU_MRR_Obj_01_02_0x690FromOutData), Bus Selector27/1  "VR_ADCU_MRR_Obj_01_02_0x690FromOutData"
  Bus Selector27/1 -> Output30/1  "<MRR_ObjDistX_01>"
  Bus Selector27/2 -> Output31/1  "<MRR_ObjRelVelX_01>"
  Bus Selector27/3 -> Switch/2  "<MRR_ObjType_01>"
  Constant/1 -> Switch/1
  Constant1/1 -> Switch/3
  Switch/1 -> ACC_Objected/1
  Bus Selector13/5 -> Out20/1  "<IPM_Line01_Type>"
  Bus Selector13/6 -> Out21/1  "<IPM_Line01_ColorClass>"
  Bus Selector13/7 -> Out22/1  "<IPM_Line01_Existence_Probability>"
  Bus Selector18/5 -> Out23/1  "<IPM_Line02_Type>"
  Bus Selector18/6 -> Out24/1  "<IPM_Line02_ColorClass>"
  Bus Selector18/7 -> Out25/1  "<IPM_Line02_Existence_Probability>"
  CCAN_ADCU_MsgFromCAN/29(CCAN_ADCU_SWM_Body_0x31AFromOutData) -> Bus Selector28/1  "CCAN_ADCU_SWM_Body_0x31AFromOutData"
  Bus Selector28/1 -> Output32/1  "<SWM_TurnIndicationAct>"
  VR_ADCU_MsgFromCAN/50(VR_ADCU_MRR_Obj_05_06_0x692FromOutData) -> Subsystem/3(VR_ADCU_MRR_Obj_05_06_0x692FromOutData)  "VR_ADCU_MRR_Obj_05_06_0x692FromOutData"
  VR_ADCU_MsgFromCAN/51(VR_ADCU_MRR_Obj_07_08_0x693FromOutData) -> Subsystem/4(VR_ADCU_MRR_Obj_07_08_0x693FromOutData)  "VR_ADCU_MRR_Obj_07_08_0x693FromOutData"
  VR_ADCU_MsgFromCAN/49(VR_ADCU_MRR_Obj_03_04_0x691FromOutData) -> Subsystem/2(VR_ADCU_MRR_Obj_03_04_0x691FromOutData)  "VR_ADCU_MRR_Obj_03_04_0x691FromOutData"
  VR_ADCU_MsgFromCAN/52(VR_ADCU_MRR_Obj_09_10_0x694FromOutData) -> Subsystem/5(VR_ADCU_MRR_Obj_09_10_0x694FromOutData)  "VR_ADCU_MRR_Obj_09_10_0x694FromOutData"
  VR_ADCU_MsgFromCAN/53(VR_ADCU_MRR_Obj_11_12_0x695FromOutData) -> Subsystem/6(VR_ADCU_MRR_Obj_11_12_0x695FromOutData)  "VR_ADCU_MRR_Obj_11_12_0x695FromOutData"
  VR_ADCU_MsgFromCAN/54(VR_ADCU_MRR_Obj_13_14_0x696FromOutData) -> Subsystem/7(VR_ADCU_MRR_Obj_13_14_0x696FromOutData)  "VR_ADCU_MRR_Obj_13_14_0x696FromOutData"
  VR_ADCU_MsgFromCAN/55(VR_ADCU_MRR_Obj_15_16_0x697FromOutData) -> Subsystem/8(VR_ADCU_MRR_Obj_15_16_0x697FromOutData)  "VR_ADCU_MRR_Obj_15_16_0x697FromOutData"
  VR_ADCU_MsgFromCAN/56(VR_ADCU_MRR_Obj_17_18_0x698FromOutData) -> Subsystem/9(VR_ADCU_MRR_Obj_17_18_0x698FromOutData)  "VR_ADCU_MRR_Obj_17_18_0x698FromOutData"
  VR_ADCU_MsgFromCAN/57(VR_ADCU_MRR_Obj_19_20_0x699FromOutData) -> Subsystem/10(VR_ADCU_MRR_Obj_19_20_0x699FromOutData)  "VR_ADCU_MRR_Obj_19_20_0x699FromOutData"
  VR_ADCU_MsgFromCAN/58(VR_ADCU_MRR_Obj_21_22_0x69AFromOutData) -> Subsystem/11(VR_ADCU_MRR_Obj_21_22_0x69AFromOutData)  "VR_ADCU_MRR_Obj_21_22_0x69AFromOutData"
  VR_ADCU_MsgFromCAN/59(VR_ADCU_MRR_Obj_23_24_0x69BFromOutData) -> Subsystem/12(VR_ADCU_MRR_Obj_23_24_0x69BFromOutData)  "VR_ADCU_MRR_Obj_23_24_0x69BFromOutData"
  VR_ADCU_MsgFromCAN/60(VR_ADCU_MRR_Obj_25_26_0x69CFromOutData) -> Subsystem/13(VR_ADCU_MRR_Obj_25_26_0x69CFromOutData)  "VR_ADCU_MRR_Obj_25_26_0x69CFromOutData"
  VR_ADCU_MsgFromCAN/61(VR_ADCU_MRR_Obj_27_28_0x69DFromOutData) -> Subsystem/14(VR_ADCU_MRR_Obj_27_28_0x69DFromOutData)  "VR_ADCU_MRR_Obj_27_28_0x69DFromOutData"
  VR_ADCU_MsgFromCAN/62(VR_ADCU_MRR_Obj_29_30_0x69EFromOutData) -> Subsystem/15(VR_ADCU_MRR_Obj_29_30_0x69EFromOutData)  "VR_ADCU_MRR_Obj_29_30_0x69EFromOutData"
  VR_ADCU_MsgFromCAN/63(VR_ADCU_MRR_Obj_31_32_0x69FFromOutData) -> Subsystem/16(VR_ADCU_MRR_Obj_31_32_0x69FFromOutData)  "VR_ADCU_MRR_Obj_31_32_0x69FFromOutData"
  Subsystem/1(1) -> Mux/1
  Subsystem/2(2) -> Mux/2
  Subsystem/3(3) -> Mux/3
  Subsystem/4(4) -> Mux/4
  Subsystem/5(5) -> Mux/5
  Subsystem/6(6) -> Mux/6
  Subsystem/7(7) -> Mux/7
  Subsystem/8(8) -> Mux/8
  Subsystem/9(9) -> Mux/9
  Subsystem/10(10) -> Mux/10
  Subsystem/11(11) -> Mux/11
  Subsystem/12(12) -> Mux/12
  Subsystem/13(13) -> Mux/13
  Subsystem/14(14) -> Mux/14
  Subsystem/15(15) -> Mux/15
  Subsystem/16(16) -> Mux/16
  Subsystem/17(17) -> Mux/17
  Subsystem/18(18) -> Mux/18
  Subsystem/19(19) -> Mux/19
  Subsystem/20(20) -> Mux/20
  Subsystem/21(21) -> Mux/21
  Subsystem/22(22) -> Mux/22
  Subsystem/23(23) -> Mux/23
  Subsystem/24(24) -> Mux/24
  Subsystem/25(25) -> Mux/25
  Subsystem/26(26) -> Mux/26
  Subsystem/27(27) -> Mux/27
  Subsystem/28(28) -> Mux/28
  Subsystem/29(29) -> Mux/29
  Subsystem/30(30) -> Mux/30
  Subsystem/31(31) -> Mux/31
  Subsystem/32(32) -> Mux/32
  Mux/1 -> MRR_obj_1_32/1
  Data Type Conversion1/1 -> Output/1
  Subsystem1/15(15) -> Mux1/15
  Subsystem1/14(14) -> Mux1/14
  Subsystem1/11(11) -> Mux1/11
  Subsystem1/10(10) -> Mux1/10
  Subsystem1/20(20) -> Mux1/20
  Subsystem1/13(13) -> Mux1/13
  Subsystem1/19(19) -> Mux1/19
  Subsystem1/5(5) -> Mux1/5
  Subsystem1/17(17) -> Mux1/17
  Subsystem1/3(3) -> Mux1/3
  VR_ADCU_MsgFromCAN/29(VR_ADCU_IPM_Obj_17_0x660FromOutData) -> Subsystem1/17(VR_ADCU_IPM_Obj_17_0x660FromOutData)  "VR_ADCU_IPM_Obj_17_0x660FromOutData"
  Subsystem1/7(7) -> Mux1/7
  Subsystem1/16(16) -> Mux1/16
  Subsystem1/4(4) -> Mux1/4
  VR_ADCU_MsgFromCAN/21(VR_ADCU_IPM_Obj_09_0x658FromOutData) -> Subsystem1/9(VR_ADCU_IPM_Obj_09_0x658FromOutData)  "VR_ADCU_IPM_Obj_09_0x658FromOutData"
  Subsystem1/18(18) -> Mux1/18
  Subsystem1/8(8) -> Mux1/8
  VR_ADCU_MsgFromCAN/17(VR_ADCU_IPM_Obj_05_0x654FromOutData) -> Subsystem1/5(VR_ADCU_IPM_Obj_05_0x654FromOutData)  "VR_ADCU_IPM_Obj_05_0x654FromOutData"
  VR_ADCU_MsgFromCAN/19(VR_ADCU_IPM_Obj_07_0x656FromOutData) -> Subsystem1/7(VR_ADCU_IPM_Obj_07_0x656FromOutData)  "VR_ADCU_IPM_Obj_07_0x656FromOutData"
  VR_ADCU_MsgFromCAN/15(VR_ADCU_IPM_Obj_03_0x652FromOutData) -> Subsystem1/3(VR_ADCU_IPM_Obj_03_0x652FromOutData)  "VR_ADCU_IPM_Obj_03_0x652FromOutData"
  Mux1/1 -> IPM_obj_1_20/1
  VR_ADCU_MsgFromCAN/28(VR_ADCU_IPM_Obj_16_0x65FFromOutData) -> Subsystem1/16(VR_ADCU_IPM_Obj_16_0x65FFromOutData)  "VR_ADCU_IPM_Obj_16_0x65FFromOutData"
  VR_ADCU_MsgFromCAN/32(VR_ADCU_IPM_Obj_20_0x663FromOutData) -> Subsystem1/20(VR_ADCU_IPM_Obj_20_0x663FromOutData)  "VR_ADCU_IPM_Obj_20_0x663FromOutData"
  VR_ADCU_MsgFromCAN/14(VR_ADCU_IPM_Obj_02_0x651FromOutData) -> Subsystem1/2(VR_ADCU_IPM_Obj_02_0x651FromOutData)  "VR_ADCU_IPM_Obj_02_0x651FromOutData"
  Subsystem1/9(9) -> Mux1/9
  Subsystem1/12(12) -> Mux1/12
  VR_ADCU_MsgFromCAN/25(VR_ADCU_IPM_Obj_13_0x65CFromOutData) -> Subsystem1/13(VR_ADCU_IPM_Obj_13_0x65CFromOutData)  "VR_ADCU_IPM_Obj_13_0x65CFromOutData"
  VR_ADCU_MsgFromCAN/18(VR_ADCU_IPM_Obj_06_0x655FromOutData) -> Subsystem1/6(VR_ADCU_IPM_Obj_06_0x655FromOutData)  "VR_ADCU_IPM_Obj_06_0x655FromOutData"
  VR_ADCU_MsgFromCAN/20(VR_ADCU_IPM_Obj_08_0x657FromOutData) -> Subsystem1/8(VR_ADCU_IPM_Obj_08_0x657FromOutData)  "VR_ADCU_IPM_Obj_08_0x657FromOutData"
  VR_ADCU_MsgFromCAN/13(VR_ADCU_IPM_Obj_01_0x650FromOutData) -> Subsystem1/1(VR_ADCU_IPM_Obj_01_0x650FromOutData)  "VR_ADCU_IPM_Obj_01_0x650FromOutData"
  VR_ADCU_MsgFromCAN/31(VR_ADCU_IPM_Obj_19_0x662FromOutData) -> Subsystem1/19(VR_ADCU_IPM_Obj_19_0x662FromOutData)  "VR_ADCU_IPM_Obj_19_0x662FromOutData"
  VR_ADCU_MsgFromCAN/30(VR_ADCU_IPM_Obj_18_0x661FromOutData) -> Subsystem1/18(VR_ADCU_IPM_Obj_18_0x661FromOutData)  "VR_ADCU_IPM_Obj_18_0x661FromOutData"
  Subsystem1/2(2) -> Mux1/2
  VR_ADCU_MsgFromCAN/16(VR_ADCU_IPM_Obj_04_0x653FromOutData) -> Subsystem1/4(VR_ADCU_IPM_Obj_04_0x653FromOutData)  "VR_ADCU_IPM_Obj_04_0x653FromOutData"
  Subsystem1/1(1) -> Mux1/1
  VR_ADCU_MsgFromCAN/26(VR_ADCU_IPM_Obj_14_0x65DFromOutData) -> Subsystem1/14(VR_ADCU_IPM_Obj_14_0x65DFromOutData)  "VR_ADCU_IPM_Obj_14_0x65DFromOutData"
  VR_ADCU_MsgFromCAN/23(VR_ADCU_IPM_Obj_11_0x65AFromOutData) -> Subsystem1/11(VR_ADCU_IPM_Obj_11_0x65AFromOutData)  "VR_ADCU_IPM_Obj_11_0x65AFromOutData"
  VR_ADCU_MsgFromCAN/24(VR_ADCU_IPM_Obj_12_0x65BFromOutData) -> Subsystem1/12(VR_ADCU_IPM_Obj_12_0x65BFromOutData)  "VR_ADCU_IPM_Obj_12_0x65BFromOutData"
  Subsystem1/6(6) -> Mux1/6
  VR_ADCU_MsgFromCAN/27(VR_ADCU_IPM_Obj_15_0x65EFromOutData) -> Subsystem1/15(VR_ADCU_IPM_Obj_15_0x65EFromOutData)  "VR_ADCU_IPM_Obj_15_0x65EFromOutData"
  VR_ADCU_MsgFromCAN/22(VR_ADCU_IPM_Obj_10_0x659FromOutData) -> Subsystem1/10(VR_ADCU_IPM_Obj_10_0x659FromOutData)  "VR_ADCU_IPM_Obj_10_0x659FromOutData"
  CCAN_ADCU_MsgFromCAN/17(CCAN_ADCU_GW_EMS_Tq_0x101FromOutData) -> Bus Selector19/1  "CCAN_ADCU_GW_EMS_Tq_0x101FromOutData"
  Bus Selector19/1 -> Output33/1  "<EMS_IndicatedRealEngTorq>"
  Bus Selector3/3 -> Out15/1  "<IPM_Line03_Existence_Probability>"
  Bus Selector4/3 -> Out16/1  "<IPM_Line04_Existence_Probability>"
  ADCU_data/12(CCAN_ADCU_GW_SRS_0x350FromInData) -> CCAN_ADCU_MsgFromCAN/25(CCAN_ADCU_GW_SRS_0x350FromInData)
  ADCU_data/10(CCAN_ADCU_GW_EMS_WhlTq_0x107FromInData) -> CCAN_ADCU_MsgFromCAN/18(CCAN_ADCU_GW_EMS_WhlTq_0x107FromInData)
  ADCU_data/9(CCAN_ADCU_GW_EMS_TqWhl_0x111FromInData) -> CCAN_ADCU_MsgFromCAN/16(CCAN_ADCU_GW_EMS_TqWhl_0x111FromInData)
  ADCU_data/1(CCAN_ADCU_ABS_Sts_0x221FromInData) -> CCAN_ADCU_MsgFromCAN/1(CCAN_ADCU_ABS_Sts_0x221FromInData)
  ADCU_data/4(CCAN_ADCU_ESP_Direction_0x235FromInData) -> CCAN_ADCU_MsgFromCAN/6(CCAN_ADCU_ESP_Direction_0x235FromInData)
  ADCU_data/17(CCAN_ADCU_ABS_Sts_0x221FromInData1) -> CCAN_ADCU_MsgFromCAN/17(CCAN_ADCU_GW_EMS_Tq_0x101FromInData)
  ADCU_data/7(CCAN_ADCU_GW_BCM_Door_0x310FromInData) -> CCAN_ADCU_MsgFromCAN/11(CCAN_ADCU_GW_BCM_Door_0x310FromInData)
  ADCU_data/5(CCAN_ADCU_ESP_Pressure_0x241FromInData) -> CCAN_ADCU_MsgFromCAN/7(CCAN_ADCU_ESP_Pressure_0x241FromInData)
  ADCU_data/16(CCAN_ADCU_SWM_MRR_0x31BFromInData) -> CCAN_ADCU_MsgFromCAN/30(CCAN_ADCU_SWM_MRR_0x31BFromInData)
  ADCU_data/8(CCAN_ADCU_GW_Body_0x321FromInData) -> CCAN_ADCU_MsgFromCAN/12(CCAN_ADCU_GW_Body_0x321FromInData)
  ADCU_data/14(CCAN_ADCU_SAS_Sensor_0x175FromInData) -> CCAN_ADCU_MsgFromCAN/27(CCAN_ADCU_SAS_Sensor_0x175FromInData)
  ADCU_data/15(CCAN_ADCU_SWM_Body_0x31AFromInData) -> CCAN_ADCU_MsgFromCAN/29(CCAN_ADCU_SWM_Body_0x31AFromInData)
  ADCU_data/3(CCAN_ADCU_ESP_AxAy_0x242FromInData) -> CCAN_ADCU_MsgFromCAN/5(CCAN_ADCU_ESP_AxAy_0x242FromInData)
  ADCU_data/6(CCAN_ADCU_ESP_Status_0x243FromInData) -> CCAN_ADCU_MsgFromCAN/9(CCAN_ADCU_ESP_Status_0x243FromInData)
  ADCU_data/13(CCAN_ADCU_GW_TCU_GearInfo_0x123FromInData) -> CCAN_ADCU_MsgFromCAN/26(CCAN_ADCU_GW_TCU_GearInfo_0x123FromInData)
  ADCU_data/11(CCAN_ADCU_GW_IC_0x510FromInData) -> CCAN_ADCU_MsgFromCAN/19(CCAN_ADCU_GW_IC_0x510FromInData)
  ADCU_data/2(CCAN_ADCU_EPS_Advanced_0x176FromInData) -> CCAN_ADCU_MsgFromCAN/3(CCAN_ADCU_EPS_Advanced_0x176FromInData)
  MRR_Obj_data/14(VR_ADCU_MRR_Obj_25_26_0x69CFromInData) -> VR_ADCU_MsgFromCAN/60(VR_ADCU_MRR_Obj_25_26_0x69CFromInData)
  IPM_Obj_data/11(VR_ADCU_IPM_Obj_10_0x659FromInData) -> VR_ADCU_MsgFromCAN/22(VR_ADCU_IPM_Obj_10_0x659FromInData)
  IPM_Obj_data/20(VR_ADCU_IPM_Obj_19_0x662FromInData) -> VR_ADCU_MsgFromCAN/31(VR_ADCU_IPM_Obj_19_0x662FromInData)
  IPM_Obj_data/19(VR_ADCU_IPM_Obj_18_0x661FromInData) -> VR_ADCU_MsgFromCAN/30(VR_ADCU_IPM_Obj_18_0x661FromInData)
  IPM_Line_data/4(VR_ADCU_IPM_Line_04_0x643FromInData) -> VR_ADCU_MsgFromCAN/9(VR_ADCU_IPM_Line_04_0x643FromInData)
  IPM_Obj_data/1(VR_ADCU_IPM_ObjHeader_0x630FromInData) -> VR_ADCU_MsgFromCAN/12(VR_ADCU_IPM_ObjHeader_0x630FromInData)
  IPM_Line_data/1(VR_ADCU_IPM_Line_01_0x640FromInData) -> VR_ADCU_MsgFromCAN/6(VR_ADCU_IPM_Line_01_0x640FromInData)
  IPM_Line_data/2(VR_ADCU_IPM_Line_02_0x641FromInData) -> VR_ADCU_MsgFromCAN/7(VR_ADCU_IPM_Line_02_0x641FromInData)
  MRR_Obj_data/11(VR_ADCU_MRR_Obj_19_20_0x699FromInData) -> VR_ADCU_MsgFromCAN/57(VR_ADCU_MRR_Obj_19_20_0x699FromInData)
  MRR_Obj_data/15(VR_ADCU_MRR_Obj_27_28_0x69DFromInData) -> VR_ADCU_MsgFromCAN/61(VR_ADCU_MRR_Obj_27_28_0x69DFromInData)
  MRR_Obj_data/10(VR_ADCU_MRR_Obj_17_18_0x698FromInData) -> VR_ADCU_MsgFromCAN/56(VR_ADCU_MRR_Obj_17_18_0x698FromInData)
  MRR_Obj_data/8(VR_ADCU_MRR_Obj_13_14_0x696FromInData) -> VR_ADCU_MsgFromCAN/54(VR_ADCU_MRR_Obj_13_14_0x696FromInData)
  MRR_Obj_data/7(VR_ADCU_MRR_Obj_11_12_0x695FromInData) -> VR_ADCU_MsgFromCAN/53(VR_ADCU_MRR_Obj_11_12_0x695FromInData)
  IPM_Obj_data/7(VR_ADCU_IPM_Obj_06_0x655FromInData) -> VR_ADCU_MsgFromCAN/18(VR_ADCU_IPM_Obj_06_0x655FromInData)
  MRR_Obj_data/16(VR_ADCU_MRR_Obj_29_30_0x69EFromInData) -> VR_ADCU_MsgFromCAN/62(VR_ADCU_MRR_Obj_29_30_0x69EFromInData)
  IPM_Obj_data/15(VR_ADCU_IPM_Obj_14_0x65DFromInData) -> VR_ADCU_MsgFromCAN/26(VR_ADCU_IPM_Obj_14_0x65DFromInData)
  IPM_Obj_data/10(VR_ADCU_IPM_Obj_09_0x658FromInData) -> VR_ADCU_MsgFromCAN/21(VR_ADCU_IPM_Obj_09_0x658FromInData)
  MRR_Obj_data/6(VR_ADCU_MRR_Obj_09_10_0x694FromInData) -> VR_ADCU_MsgFromCAN/52(VR_ADCU_MRR_Obj_09_10_0x694FromInData)
  IPM_Obj_data/3(VR_ADCU_IPM_Obj_02_0x651FromInData) -> VR_ADCU_MsgFromCAN/14(VR_ADCU_IPM_Obj_02_0x651FromInData)
  MRR_Obj_data/9(VR_ADCU_MRR_Obj_15_16_0x697FromInData) -> VR_ADCU_MsgFromCAN/55(VR_ADCU_MRR_Obj_15_16_0x697FromInData)
  IPM_Obj_data/16(VR_ADCU_IPM_Obj_15_0x65EFromInData) -> VR_ADCU_MsgFromCAN/27(VR_ADCU_IPM_Obj_15_0x65EFromInData)
  IPM_Obj_data/13(VR_ADCU_IPM_Obj_12_0x65BFromInData) -> VR_ADCU_MsgFromCAN/24(VR_ADCU_IPM_Obj_12_0x65BFromInData)
  IPM_Obj_data/9(VR_ADCU_IPM_Obj_08_0x657FromInData) -> VR_ADCU_MsgFromCAN/20(VR_ADCU_IPM_Obj_08_0x657FromInData)
  IPM_Obj_data/8(VR_ADCU_IPM_Obj_07_0x656FromInData) -> VR_ADCU_MsgFromCAN/19(VR_ADCU_IPM_Obj_07_0x656FromInData)
  IPM_Obj_data/6(VR_ADCU_IPM_Obj_05_0x654FromInData) -> VR_ADCU_MsgFromCAN/17(VR_ADCU_IPM_Obj_05_0x654FromInData)
  MRR_Obj_data/5(VR_ADCU_MRR_Obj_07_08_0x693FromInData) -> VR_ADCU_MsgFromCAN/51(VR_ADCU_MRR_Obj_07_08_0x693FromInData)
  MRR_Obj_data/12(VR_ADCU_MRR_Obj_21_22_0x69AFromInData) -> VR_ADCU_MsgFromCAN/58(VR_ADCU_MRR_Obj_21_22_0x69AFromInData)
  IPM_Obj_data/14(VR_ADCU_IPM_Obj_13_0x65CFromInData) -> VR_ADCU_MsgFromCAN/25(VR_ADCU_IPM_Obj_13_0x65CFromInData)
  MRR_Obj_data/1(VR_ADCU_MRR_ObjHeader_0x680FromInData) -> VR_ADCU_MsgFromCAN/47(VR_ADCU_MRR_ObjHeader_0x680FromInData)
  IPM_Obj_data/21(VR_ADCU_IPM_Obj_20_0x663FromInData) -> VR_ADCU_MsgFromCAN/32(VR_ADCU_IPM_Obj_20_0x663FromInData)
  IPM_Obj_data/18(VR_ADCU_IPM_Obj_17_0x660FromInData) -> VR_ADCU_MsgFromCAN/29(VR_ADCU_IPM_Obj_17_0x660FromInData)
  IPM_Obj_data/4(VR_ADCU_IPM_Obj_03_0x652FromInData) -> VR_ADCU_MsgFromCAN/15(VR_ADCU_IPM_Obj_03_0x652FromInData)
  MRR_Obj_data/2(VR_ADCU_MRR_Obj_01_02_0x690FromInData) -> VR_ADCU_MsgFromCAN/48(VR_ADCU_MRR_Obj_01_02_0x690FromInData)
  MRR_Obj_data/3(VR_ADCU_MRR_Obj_03_04_0x691FromInData) -> VR_ADCU_MsgFromCAN/49(VR_ADCU_MRR_Obj_03_04_0x691FromInData)
  IPM_Obj_data/5(VR_ADCU_IPM_Obj_04_0x653FromInData) -> VR_ADCU_MsgFromCAN/16(VR_ADCU_IPM_Obj_04_0x653FromInData)
  IPM_Obj_data/12(VR_ADCU_IPM_Obj_11_0x65AFromInData) -> VR_ADCU_MsgFromCAN/23(VR_ADCU_IPM_Obj_11_0x65AFromInData)
  IPM_Line_data/3(VR_ADCU_IPM_Line_03_0x642FromInData) -> VR_ADCU_MsgFromCAN/8(VR_ADCU_IPM_Line_03_0x642FromInData)
  IPM_Obj_data/2(VR_ADCU_IPM_Obj_01_0x650FromInData) -> VR_ADCU_MsgFromCAN/13(VR_ADCU_IPM_Obj_01_0x650FromInData)
  MRR_Obj_data/13(VR_ADCU_MRR_Obj_23_24_0x69BFromInData) -> VR_ADCU_MsgFromCAN/59(VR_ADCU_MRR_Obj_23_24_0x69BFromInData)
  IPM_Obj_data/17(VR_ADCU_IPM_Obj_16_0x65FFromInData) -> VR_ADCU_MsgFromCAN/28(VR_ADCU_IPM_Obj_16_0x65FFromInData)
  MRR_Obj_data/17(VR_ADCU_MRR_Obj_31_32_0x69FFromInData) -> VR_ADCU_MsgFromCAN/63(VR_ADCU_MRR_Obj_31_32_0x69FFromInData)
  MRR_Obj_data/4(VR_ADCU_MRR_Obj_05_06_0x692FromInData) -> VR_ADCU_MsgFromCAN/50(VR_ADCU_MRR_Obj_05_06_0x692FromInData)
